simulink model "diagrama_completo"  (R2020b)
settings: Solver=VariableStepAuto  StartTime=0.0  StopTime=25  MaxStep=1e-4  RelTol=1e-4
model workspace (MAT data in the model file):
  Cts = 0.818
  Jeq = 5.65099476805e-06
  Ld = 0.0066
  Lls = 0.0008
  Lq = 0.0058
  Pp = 3
  Rs = 1.02
  Rts_amb = 146.7
  beq = 1.5e-05
  lambda_m = 0.01546
  r = 314.3008
  ws = 15000
  wsv = 30000
values from neighbouring files (symbols this model uses):
  ba = Jeq*n*wpos    (= 0.0113019895361)    [valores.m]
  kotheta = 3*pobs    (= 9600)    [valores.m]
  koTl = (pobs^3)    (= 32768000000)    [valores.m]
  kow = 3*(pobs^2)    (= 30720000)    [valores.m]
  ksa = ba*wpos    (= 9.04159162887)    [valores.m]
  ksia = ksa*wint    (= 2893.30932124)    [valores.m]
  R0 = Lls*pi    (= 4)    [valores.m]
  Rd = Ld*pi    (= 33)    [valores.m]
  Rq = Lq*pi    (= 29)    [valores.m]
undefined symbols (not defined in the file or in its folder): sigbuilder_block
(part 1 of 2)
settings Model: Creator=Matias  LastModifiedBy=Matias

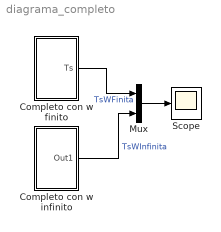
== system diagrama_completo ==
  Completo con w finito : Subsystem
  Completo con w infinito : Subsystem
  Mux : Mux  Inputs=2
  Scope : Scope
  wires:
  Completo con w finito/1(Ts) -> Mux/1  "TsWFinita"
  Completo con w infinito/1(Out1) -> Mux/2  "TsWInfinita"
  Mux/1 -> Scope/1

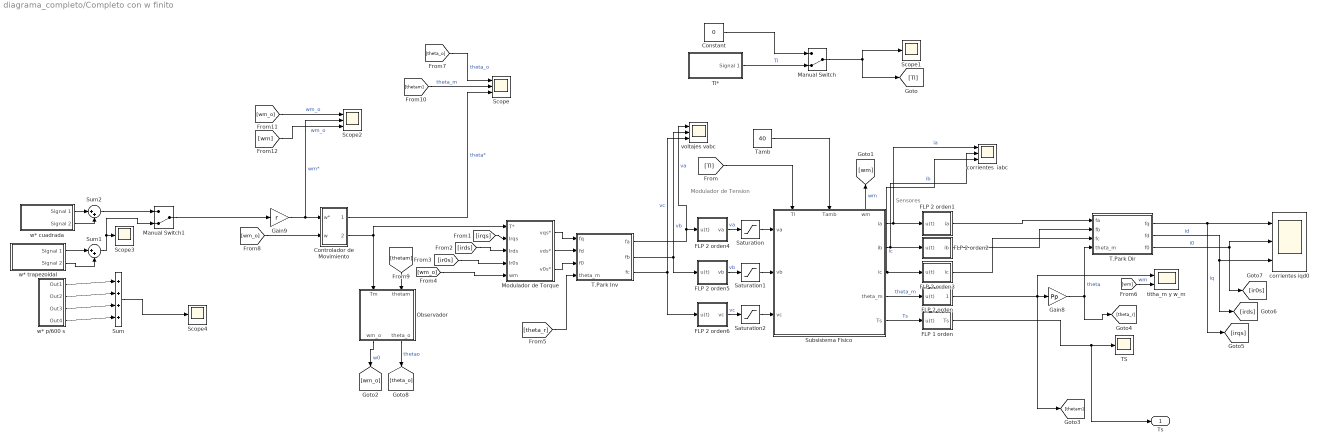
== system diagrama_completo/Completo con w finito ==
  note: Sensores
  note: Modulador de Tension
  Constant : Constant  Value=0
  Controlador de Movimiento : Subsystem
  FLP 1 orden : Subsystem
  FLP 2 orden : Subsystem
  FLP 2 orden1 : Subsystem
  FLP 2 orden2 : Subsystem
  FLP 2 orden3 : Subsystem
  FLP 2 orden4 : Subsystem
  FLP 2 orden5 : Subsystem
  FLP 2 orden6 : Subsystem
  Gain8 : Gain  Gain=Pp
  Gain9 : Gain  Gain=r
  Manual Switch : ManualSwitch  CurrentSetting=0
  Manual Switch1 : ManualSwitch  CurrentSetting=0
  Modulador de Torque : Subsystem
  Observador : Subsystem
  Saturation : Saturate  UpperLimit=19.59  LowerLimit=-19.59
  Saturation1 : Saturate  UpperLimit=19.59  LowerLimit=-19.59
  Saturation2 : Saturate  UpperLimit=19.59  LowerLimit=-19.59
  Scope : Scope  NumInputPorts=3
  Scope1 : Scope
  Scope2 : Scope  NumInputPorts=3
  Scope3 : Scope
  Scope4 : Scope
  Subsistema Fisico : Subsystem
      settings: PortSchema="{\"entries\":[{\"content\":{\"sides\":[{\"content\":{\"connectorIds\":[\"In1\",\"In2\",\"In3\"]},\"type\":\"ConnectorPlacement.EquallySpacedRectSide\",\"uuid\":\"428e53fe-c6d6-4999-95eb-db171c1d7752\"},{\"content\":{\"connectorIds\":[\"Out1\",\"Out2\",\"Out3\",\"Out4\",\"Out5\"],\"side\":\"RIGHT\"},\"type\":\"ConnectorPlacement.EquallySpacedRectSide\",\"uuid\":\"d3984cce-d898-4b9d-ab92-7967eebad5db\"},{\"content\":{\"connectorIds\":[\"In4\",\"In5\",\"Out6\"],\"side\":\"TOP\"},\"type\":\"ConnectorPlacement.EquallySpacedRectSide\",\"uuid\":\"4e08f4f3-ce82-4568-8c70-e26e1ed2ccd9\"},{\"content\":{\"connectorIds\":[],\"side\":\"BOTTOM\"},\"type\":\"ConnectorPlacement.EquallySpacedRectSide\",\"uuid\":\"f5359b7b-31c8-439d-9b4b-495d60398ac6\"},{\"content\":{\"connectorIds\":[],\"side\":\"HIDDEN\"},\"type\":\"ConnectorPlacement.EquallySpacedRectSide\",\"uuid\":\"fe5ef39c-0012-48bd-8627-0cf1abf153f6\"}]},\"type\":\"ConnectorPlacement.EquallySpacedConnector\",\"uuid\":\"3b2746a1-6d8c-49ea-8ba7-7e2e359e7a22\"}],\"packageUris\":[\"http://schema.mathworks.com/mf0/Connector/R2020b\"],\"version\":\"1.0\"}"
  Sum : Sum  Inputs=|+|+|+|+
  Sum1 : Sum  Inputs=|++
  Sum2 : Sum  Inputs=|++
  T.Park Dir : MATLAB Function  TreatAsAtomicUnit=on
  T.Park Inv : MATLAB Function  TreatAsAtomicUnit=on
  TS : Scope
  Tamb : Constant  Value=40
  Tl* : Subsystem  Tag=STV Subsys  LoadFcn=sigbuilder_block('load');  StartFcn=sigbuilder_block('start');  StopFcn=sigbuilder_block('stop');  ClipboardFcn=sigbuilder_block('clipboard');  mask(Sigbuilder block){tuvar=[0:10]}
      mask help: Simulink:masks:SigbuilderBlock_MD
      mask init:
      | if ~strcmp(get_param(bdroot(gcbh),'SimulationStatus'),'stopped') tuvar = sigbuilder_block('maskInit'); end
      settings: CopyFcn=sigbuilder_block('copy');  DeleteFcn=sigbuilder_block('delete');  ModelCloseFcn=sigbuilder_block('modelClose');  PreSaveFcn=sigbuilder_block('preSave');  PauseFcn=sigbuilder_block('pause');  ContinueFcn=sigbuilder_block('continue');  NameChangeFcn=sigbuilder_block('namechange');  OpenFcn=sigbuilder_block('open',[388.2 64.2 550.8 400.2 ]);  CloseFcn=sigbuilder_block('close');
      mask Display: plot(0, 0, 100, 100,[2, 2, 32, 32, 2], [68, 8, 8, 68, 68],[32, 2], [38, 38], [32, 19, 2],[53, 60, 44], [32, 17, 17, 2],[16, 16, 31, 31]);txt = getActiveGroup(gcbh);text(2, 100, txt,'verticalAlignment', 'top');
  corrientes  iabc : Scope  NumInputPorts=3
  corrientes iqd0 : Scope  NumInputPorts=3
  titha_m y w_m : Scope  NumInputPorts=2
  voltajes vabc : Scope  NumInputPorts=3
  w* cuadrada : Subsystem  Tag=STV Subsys  LoadFcn=sigbuilder_block('load');  StartFcn=sigbuilder_block('start');  StopFcn=sigbuilder_block('stop');  ClipboardFcn=sigbuilder_block('clipboard');  mask(Sigbuilder block){tuvar=[0:10]}
      mask help: Simulink:masks:SigbuilderBlock_MD
      mask init:
      | if ~strcmp(get_param(bdroot(gcbh),'SimulationStatus'),'stopped') tuvar = sigbuilder_block('maskInit'); end
      settings: CopyFcn=sigbuilder_block('copy');  DeleteFcn=sigbuilder_block('delete');  ModelCloseFcn=sigbuilder_block('modelClose');  PreSaveFcn=sigbuilder_block('preSave');  PauseFcn=sigbuilder_block('pause');  ContinueFcn=sigbuilder_block('continue');  NameChangeFcn=sigbuilder_block('namechange');  OpenFcn=sigbuilder_block('open',[5.4 36 1141.2 516.6 ]);  CloseFcn=sigbuilder_block('close');
      mask Display: plot(0, 0, 100, 100,[2, 2, 32, 32, 2], [68, 8, 8, 68, 68],[32, 2], [38, 38], [32, 19, 2],[53, 60, 44], [32, 17, 17, 2],[16, 16, 31, 31]);txt = getActiveGroup(gcbh);text(2, 100, txt,'verticalAlignment', 'top');
  w* p/600 s : Subsystem
  w* trapezoidal : Subsystem  Tag=STV Subsys  LoadFcn=sigbuilder_block('load');  StartFcn=sigbuilder_block('start');  StopFcn=sigbuilder_block('stop');  ClipboardFcn=sigbuilder_block('clipboard');  mask(Sigbuilder block){tuvar=[0:10]}
      mask help: Simulink:masks:SigbuilderBlock_MD
      mask init:
      | if ~strcmp(get_param(bdroot(gcbh),'SimulationStatus'),'stopped') tuvar = sigbuilder_block('maskInit'); end
      settings: CopyFcn=sigbuilder_block('copy');  DeleteFcn=sigbuilder_block('delete');  ModelCloseFcn=sigbuilder_block('modelClose');  PreSaveFcn=sigbuilder_block('preSave');  PauseFcn=sigbuilder_block('pause');  ContinueFcn=sigbuilder_block('continue');  NameChangeFcn=sigbuilder_block('namechange');  OpenFcn=sigbuilder_block('open',[5.4 36 1141.2 516.6 ]);  CloseFcn=sigbuilder_block('close');
      mask Display: plot(0, 0, 100, 100,[2, 2, 32, 32, 2], [68, 8, 8, 68, 68],[32, 2], [38, 38], [32, 19, 2],[53, 60, 44], [32, 17, 17, 2],[16, 16, 31, 31]);txt = getActiveGroup(gcbh);text(2, 100, txt,'verticalAlignment', 'top');
  Ts : Outport
  wires:
  T.Park Dir/2(fd) -> [irds], corrientes iqd0/3  "id"
  Modulador de Torque/2(vds*) -> T.Park Inv/2(fd)
  Subsistema Fisico/2(ib) -> FLP 2 orden2/1(u(t)), corrientes  iabc/2  "ib"
  FLP 2 orden6/1(vc) -> Saturation2/1  "vc"
  Gain8/1 -> T.Park Dir/4(theta_m), [theta_r]  "theta"
  Saturation1/1 -> Subsistema Fisico/2(vb)
  [thetam] -> Observador/2(thetam)
  [wm_o] -> Modulador de Torque/5(wm)
  Saturation/1 -> Subsistema Fisico/1(va)
  Sum/1 -> Scope4/1
  w* cuadrada/1(Signal 1) -> Sum2/1
  Subsistema Fisico/3(ic) -> FLP 2 orden3/1(u(t)), corrientes  iabc/3  "ic"
  FLP 2 orden4/1(va) -> Saturation/1  "va"
  w* p/600 s/2(Out2) -> Sum/2
  Subsistema Fisico/5(Ts) -> FLP 1 orden/1(u(t))  "Ts"
  T.Park Inv/1(fa) -> FLP 2 orden4/1(u(t)), voltajes vabc/1  "va"
  Manual Switch1/1 -> Gain9/1
  FLP 2 orden/1(theta) -> [thetam], titha_m y w_m/1, Gain8/1
  Tl*/1(Signal 1) -> Manual Switch/2  "Tl"
  Modulador de Torque/1(vqs*) -> T.Park Inv/1(fq)
  Saturation2/1 -> Subsistema Fisico/3(vc)
  w* trapezoidal/1(Signal 1) -> Sum1/1
  [irqs] -> Modulador de Torque/2(Irqs)
  Subsistema Fisico/1(ia) -> corrientes  iabc/1, FLP 2 orden1/1(u(t))  "ia"
  Sum1/1 -> Manual Switch1/2, Scope3/1
  FLP 2 orden2/1(ib) -> T.Park Dir/2(fb)
  [irds] -> Modulador de Torque/3(Irds)
  Tamb/1 -> Subsistema Fisico/5(Tamb)
  Constant/1 -> Manual Switch/1
  [theta_r] -> T.Park Inv/4(theta_m)
  T.Park Dir/1(fq) -> [irqs], corrientes iqd0/1  "iq"
  [ir0s] -> Modulador de Torque/4(Ir0s)
  [wm_o] -> Scope2/1  "wm_o"
  Subsistema Fisico/4(theta_m) -> FLP 2 orden/1(u(t))  "theta_m"
  [wm_o] -> Controlador de Movimiento/2(w)
  [Tl] -> Subsistema Fisico/4(Tl)
  T.Park Dir/3(f0) -> [ir0s], corrientes iqd0/2  "i0"
  Sum2/1 -> Manual Switch1/1
  Observador/1(wm_o) -> [wm_o]  "w0"
  w* p/600 s/1(Out1) -> Sum/1
  [wm] -> titha_m y w_m/2  "wm"
  Gain9/1 -> Scope2/2, Controlador de Movimiento/1(w*)  "wm*"
  Observador/2(theta_o) -> [theta_o]  "thetao"
  Controlador de Movimiento/1(Theta*) -> Scope/3  "theta*"
  w* trapezoidal/2(Signal 2) -> Sum1/2
  [theta_o] -> Scope/1  "theta_o"
  Manual Switch/1 -> [Tl], Scope1/1
  [thetam] -> Scope/2  "theta_m"
  Subsistema Fisico/6(wm) -> [wm]  "wm"
  Modulador de Torque/3(v0s*) -> T.Park Inv/3(f0)
  FLP 2 orden3/1(ic) -> T.Park Dir/3(fc)
  w* p/600 s/3(Out3) -> Sum/3
  FLP 1 orden/1(Ts) -> Ts/1, TS/1
  Controlador de Movimiento/2(Tm*') -> Modulador de Torque/1(T*), Observador/1(Tm)
  w* cuadrada/2(Signal 2) -> Sum2/2
  T.Park Inv/3(fc) -> voltajes vabc/3, FLP 2 orden6/1(u(t))  "vc"
  T.Park Inv/2(fb) -> FLP 2 orden5/1(u(t)), voltajes vabc/2  "vb"
  FLP 2 orden1/1(ia) -> T.Park Dir/1(fa)
  w* p/600 s/4(Out4) -> Sum/4
  [wm] -> Scope2/3  "wm_o"
  FLP 2 orden5/1(vb) -> Saturation1/1  "vb"

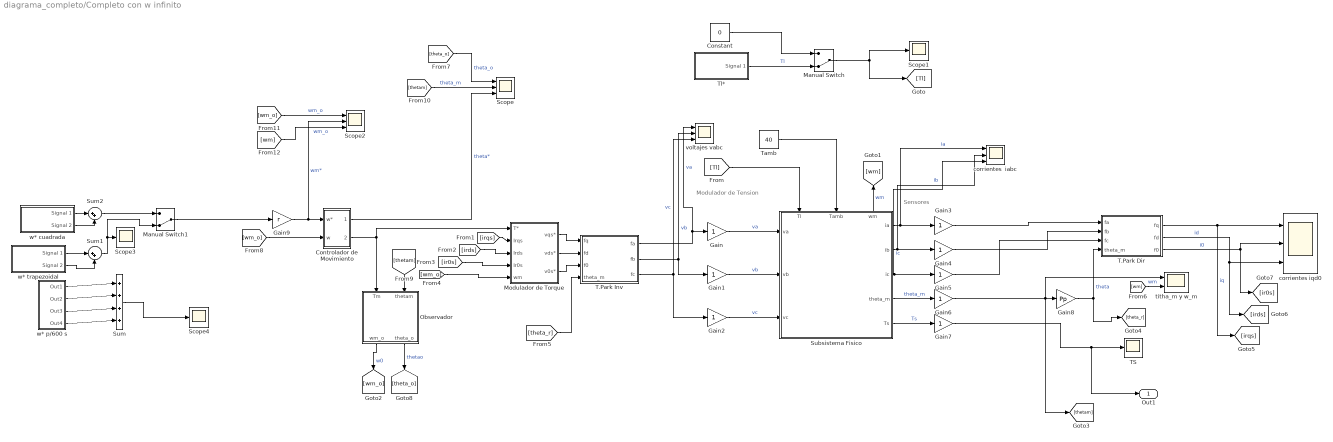
== system diagrama_completo/Completo con w infinito ==
  note: Sensores
  note: Modulador de Tension
  Constant : Constant  Value=0
  Controlador de Movimiento : Subsystem
  Gain{,1..7} (8 alike) : Gain
  Gain8 : Gain  Gain=Pp
  Gain9 : Gain  Gain=r
  Manual Switch : ManualSwitch  CurrentSetting=0
  Manual Switch1 : ManualSwitch  CurrentSetting=0
  Modulador de Torque : Subsystem
  Observador : Subsystem
  Scope : Scope  NumInputPorts=3
  Scope1 : Scope
  Scope2 : Scope  NumInputPorts=3
  Scope3 : Scope
  Scope4 : Scope
  Subsistema Fisico : Subsystem
      settings: PortSchema="{\"entries\":[{\"content\":{\"sides\":[{\"content\":{\"connectorIds\":[\"In1\",\"In2\",\"In3\"]},\"type\":\"ConnectorPlacement.EquallySpacedRectSide\",\"uuid\":\"428e53fe-c6d6-4999-95eb-db171c1d7752\"},{\"content\":{\"connectorIds\":[\"Out1\",\"Out2\",\"Out3\",\"Out4\",\"Out5\"],\"side\":\"RIGHT\"},\"type\":\"ConnectorPlacement.EquallySpacedRectSide\",\"uuid\":\"d3984cce-d898-4b9d-ab92-7967eebad5db\"},{\"content\":{\"connectorIds\":[\"In4\",\"In5\",\"Out6\"],\"side\":\"TOP\"},\"type\":\"ConnectorPlacement.EquallySpacedRectSide\",\"uuid\":\"4e08f4f3-ce82-4568-8c70-e26e1ed2ccd9\"},{\"content\":{\"connectorIds\":[],\"side\":\"BOTTOM\"},\"type\":\"ConnectorPlacement.EquallySpacedRectSide\",\"uuid\":\"f5359b7b-31c8-439d-9b4b-495d60398ac6\"},{\"content\":{\"connectorIds\":[],\"side\":\"HIDDEN\"},\"type\":\"ConnectorPlacement.EquallySpacedRectSide\",\"uuid\":\"fe5ef39c-0012-48bd-8627-0cf1abf153f6\"}]},\"type\":\"ConnectorPlacement.EquallySpacedConnector\",\"uuid\":\"3b2746a1-6d8c-49ea-8ba7-7e2e359e7a22\"}],\"packageUris\":[\"http://schema.mathworks.com/mf0/Connector/R2020b\"],\"version\":\"1.0\"}"
  Sum : Sum  Inputs=|+|+|+|+
  Sum1 : Sum  Inputs=|++
  Sum2 : Sum  Inputs=|++
  T.Park Dir : MATLAB Function  TreatAsAtomicUnit=on
  T.Park Inv : MATLAB Function  TreatAsAtomicUnit=on
  TS : Scope
  Tamb : Constant  Value=40
  Tl* : Subsystem  Tag=STV Subsys  LoadFcn=sigbuilder_block('load');  StartFcn=sigbuilder_block('start');  StopFcn=sigbuilder_block('stop');  ClipboardFcn=sigbuilder_block('clipboard');  mask(Sigbuilder block){tuvar=[0:10]}
      mask help: Simulink:masks:SigbuilderBlock_MD
      mask init:
      | if ~strcmp(get_param(bdroot(gcbh),'SimulationStatus'),'stopped') tuvar = sigbuilder_block('maskInit'); end
      settings: CopyFcn=sigbuilder_block('copy');  DeleteFcn=sigbuilder_block('delete');  ModelCloseFcn=sigbuilder_block('modelClose');  PreSaveFcn=sigbuilder_block('preSave');  PauseFcn=sigbuilder_block('pause');  ContinueFcn=sigbuilder_block('continue');  NameChangeFcn=sigbuilder_block('namechange');  OpenFcn=sigbuilder_block('open',[388.2 64.2 550.8 400.2 ]);  CloseFcn=sigbuilder_block('close');
      mask Display: plot(0, 0, 100, 100,[2, 2, 32, 32, 2], [68, 8, 8, 68, 68],[32, 2], [38, 38], [32, 19, 2],[53, 60, 44], [32, 17, 17, 2],[16, 16, 31, 31]);txt = getActiveGroup(gcbh);text(2, 100, txt,'verticalAlignment', 'top');
  corrientes  iabc : Scope  NumInputPorts=3
  corrientes iqd0 : Scope  NumInputPorts=3
  titha_m y w_m : Scope  NumInputPorts=2
  voltajes vabc : Scope  NumInputPorts=3
  w* cuadrada : Subsystem  Tag=STV Subsys  LoadFcn=sigbuilder_block('load');  StartFcn=sigbuilder_block('start');  StopFcn=sigbuilder_block('stop');  ClipboardFcn=sigbuilder_block('clipboard');  mask(Sigbuilder block){tuvar=[0:10]}
      mask help: Simulink:masks:SigbuilderBlock_MD
      mask init:
      | if ~strcmp(get_param(bdroot(gcbh),'SimulationStatus'),'stopped') tuvar = sigbuilder_block('maskInit'); end
      settings: CopyFcn=sigbuilder_block('copy');  DeleteFcn=sigbuilder_block('delete');  ModelCloseFcn=sigbuilder_block('modelClose');  PreSaveFcn=sigbuilder_block('preSave');  PauseFcn=sigbuilder_block('pause');  ContinueFcn=sigbuilder_block('continue');  NameChangeFcn=sigbuilder_block('namechange');  OpenFcn=sigbuilder_block('open',[5.4 36 1141.2 516.6 ]);  CloseFcn=sigbuilder_block('close');
      mask Display: plot(0, 0, 100, 100,[2, 2, 32, 32, 2], [68, 8, 8, 68, 68],[32, 2], [38, 38], [32, 19, 2],[53, 60, 44], [32, 17, 17, 2],[16, 16, 31, 31]);txt = getActiveGroup(gcbh);text(2, 100, txt,'verticalAlignment', 'top');
  w* p/600 s : Subsystem
  w* trapezoidal : Subsystem  Tag=STV Subsys  LoadFcn=sigbuilder_block('load');  StartFcn=sigbuilder_block('start');  StopFcn=sigbuilder_block('stop');  ClipboardFcn=sigbuilder_block('clipboard');  mask(Sigbuilder block){tuvar=[0:10]}
      mask help: Simulink:masks:SigbuilderBlock_MD
      mask init:
      | if ~strcmp(get_param(bdroot(gcbh),'SimulationStatus'),'stopped') tuvar = sigbuilder_block('maskInit'); end
      settings: CopyFcn=sigbuilder_block('copy');  DeleteFcn=sigbuilder_block('delete');  ModelCloseFcn=sigbuilder_block('modelClose');  PreSaveFcn=sigbuilder_block('preSave');  PauseFcn=sigbuilder_block('pause');  ContinueFcn=sigbuilder_block('continue');  NameChangeFcn=sigbuilder_block('namechange');  OpenFcn=sigbuilder_block('open',[5.4 36 1141.2 516.6 ]);  CloseFcn=sigbuilder_block('close');
      mask Display: plot(0, 0, 100, 100,[2, 2, 32, 32, 2], [68, 8, 8, 68, 68],[32, 2], [38, 38], [32, 19, 2],[53, 60, 44], [32, 17, 17, 2],[16, 16, 31, 31]);txt = getActiveGroup(gcbh);text(2, 100, txt,'verticalAlignment', 'top');
  Out1 : Outport
  wires:
  [theta_r] -> T.Park Inv/4(theta_m)
  w* p/600 s/4(Out4) -> Sum/4
  [wm_o] -> Controlador de Movimiento/2(w)
  Gain8/1 -> T.Park Dir/4(theta_m), [theta_r]  "theta"
  Manual Switch1/1 -> Gain9/1
  Controlador de Movimiento/1(Theta*) -> Scope/3  "theta*"
  Subsistema Fisico/3(ic) -> Gain5/1, corrientes  iabc/3  "ic"
  T.Park Dir/1(fq) -> [irqs], corrientes iqd0/1  "iq"
  Gain/1 -> Subsistema Fisico/1(va)  "va"
  T.Park Inv/2(fb) -> Gain1/1, voltajes vabc/2  "vb"
  Subsistema Fisico/2(ib) -> Gain4/1, corrientes  iabc/2  "ib"
  Gain6/1 -> [thetam], titha_m y w_m/1, Gain8/1
  w* cuadrada/2(Signal 2) -> Sum2/2
  T.Park Inv/1(fa) -> Gain/1, voltajes vabc/1  "va"
  T.Park Dir/2(fd) -> [irds], corrientes iqd0/3  "id"
  Modulador de Torque/1(vqs*) -> T.Park Inv/1(fq)
  Modulador de Torque/3(v0s*) -> T.Park Inv/3(f0)
  Gain3/1 -> T.Park Dir/1(fa)
  Observador/2(theta_o) -> [theta_o]  "thetao"
  Gain7/1 -> Out1/1, TS/1
  Subsistema Fisico/4(theta_m) -> Gain6/1  "theta_m"
  Controlador de Movimiento/2(Tm*') -> Modulador de Torque/1(T*), Observador/1(Tm)
  w* p/600 s/2(Out2) -> Sum/2
  Gain9/1 -> Scope2/2, Controlador de Movimiento/1(w*)  "wm*"
  Sum1/1 -> Manual Switch1/2, Scope3/1
  [theta_o] -> Scope/1  "theta_o"
  [Tl] -> Subsistema Fisico/4(Tl)
  [thetam] -> Scope/2  "theta_m"
  w* p/600 s/1(Out1) -> Sum/1
  w* trapezoidal/1(Signal 1) -> Sum1/1
  w* cuadrada/1(Signal 1) -> Sum2/1
  Tl*/1(Signal 1) -> Manual Switch/2  "Tl"
  T.Park Dir/3(f0) -> [ir0s], corrientes iqd0/2  "i0"
  w* p/600 s/3(Out3) -> Sum/3
  Gain5/1 -> T.Park Dir/3(fc)
  Gain2/1 -> Subsistema Fisico/3(vc)  "vc"
  [irqs] -> Modulador de Torque/2(Irqs)
  T.Park Inv/3(fc) -> Gain2/1, voltajes vabc/3  "vc"
  [wm_o] -> Modulador de Torque/5(wm)
  [irds] -> Modulador de Torque/3(Irds)
  [thetam] -> Observador/2(thetam)
  [wm] -> Scope2/3  "wm_o"
  Subsistema Fisico/6(wm) -> [wm]  "wm"
  Sum2/1 -> Manual Switch1/1
  [wm] -> titha_m y w_m/2  "wm"
  w* trapezoidal/2(Signal 2) -> Sum1/2
  Manual Switch/1 -> [Tl], Scope1/1
  Constant/1 -> Manual Switch/1
  Sum/1 -> Scope4/1
  Subsistema Fisico/5(Ts) -> Gain7/1  "Ts"
  Subsistema Fisico/1(ia) -> Gain3/1, corrientes  iabc/1  "ia"
  Tamb/1 -> Subsistema Fisico/5(Tamb)
  [ir0s] -> Modulador de Torque/4(Ir0s)
  Modulador de Torque/2(vds*) -> T.Park Inv/2(fd)
  Gain4/1 -> T.Park Dir/2(fb)
  Gain1/1 -> Subsistema Fisico/2(vb)  "vb"
  Observador/1(wm_o) -> [wm_o]  "w0"
  [wm_o] -> Scope2/1  "wm_o"

== system diagrama_completo/Completo con w finito/Controlador de Movimiento ==
  w* : Inport
  w : Inport  Port=2
  Gain : Gain  Gain=ba
  Gain1 : Gain  Gain=ksa
  Gain2 : Gain  Gain=ksia
  Integrator : Integrator
  Integrator1 : Integrator
  Integrator2 : Integrator
  Sum : Sum  Inputs=|+++
  Sum1 : Sum  Inputs=|+-
  Theta* : Outport
  Tm*' : Outport  Port=2
  wires:
  w*/1 -> Integrator2/1, Sum1/1
  w/1 -> Sum1/2
  Sum1/1 -> Integrator/1, Gain/1  "ew"
  Sum/1 -> Tm*'/1
  Gain/1 -> Sum/3
  Gain1/1 -> Sum/2
  Integrator1/1 -> Gain2/1  "etheta/s"
  Integrator/1 -> Integrator1/1, Gain1/1  "etheta"
  Gain2/1 -> Sum/1
  Integrator2/1 -> Theta*/1  "etheta"

== system diagrama_completo/Completo con w finito/FLP 1 orden ==
  u(t) : Inport
  Gain : Gain
  Gain1 : Gain
  Gain2 : Gain  Gain=1/2
  Integrator1 : Integrator  InitialCondition=40
  Sum : Sum  Inputs=|+|-
  Ts : Outport
  wires:
  u(t)/1 -> Gain/1
  Integrator1/1 -> Ts/1, Gain1/1  "x1"
  Gain/1 -> Sum/1
  Gain1/1 -> Sum/2
  Sum/1 -> Gain2/1  "d(x1)"
  Gain2/1 -> Integrator1/1

== system diagrama_completo/Completo con w finito/FLP 2 orden ==
  u(t) : Inport
  Gain : Gain  Gain=ws^2
  Gain1 : Gain  Gain=2*ws*1
  Gain2 : Gain  Gain=(ws^2)
  Integrator : Integrator
  Integrator1 : Integrator
  Sum : Sum  Inputs=|+|-|-
  theta : Outport
  wires:
  u(t)/1 -> Gain/1
  Integrator1/1 -> Gain1/1, Integrator/1  "x2"
  Integrator/1 -> Gain2/1, theta/1  "x1"
  Gain/1 -> Sum/1
  Sum/1 -> Integrator1/1  "d(x2)"
  Gain1/1 -> Sum/3
  Gain2/1 -> Sum/2

== system diagrama_completo/Completo con w finito/FLP 2 orden1 ==
  u(t) : Inport
  Gain : Gain  Gain=ws^2
  Gain1 : Gain  Gain=2*ws*1
  Gain2 : Gain  Gain=(ws^2)
  Integrator : Integrator
  Integrator1 : Integrator
  Sum : Sum  Inputs=|+|-|-
  ia : Outport
  wires:
  u(t)/1 -> Gain/1
  Integrator1/1 -> Gain1/1, Integrator/1  "x2"
  Integrator/1 -> Gain2/1, ia/1  "x1"
  Gain/1 -> Sum/1
  Sum/1 -> Integrator1/1  "d(x2)"
  Gain1/1 -> Sum/3
  Gain2/1 -> Sum/2

== system diagrama_completo/Completo con w finito/FLP 2 orden2 ==
  u(t) : Inport
  Gain : Gain  Gain=ws^2
  Gain1 : Gain  Gain=2*ws*1
  Gain2 : Gain  Gain=(ws^2)
  Integrator : Integrator
  Integrator1 : Integrator
  Sum : Sum  Inputs=|+|-|-
  ib : Outport
  wires:
  u(t)/1 -> Gain/1
  Integrator1/1 -> Gain1/1, Integrator/1  "x2"
  Integrator/1 -> Gain2/1, ib/1  "x1"
  Gain/1 -> Sum/1
  Sum/1 -> Integrator1/1  "d(x2)"
  Gain1/1 -> Sum/3
  Gain2/1 -> Sum/2

== system diagrama_completo/Completo con w finito/FLP 2 orden3 ==
  u(t) : Inport
  Gain : Gain  Gain=ws^2
  Gain1 : Gain  Gain=2*ws*1
  Gain2 : Gain  Gain=(ws^2)
  Integrator : Integrator
  Integrator1 : Integrator
  Sum : Sum  Inputs=|+|-|-
  ic : Outport
  wires:
  u(t)/1 -> Gain/1
  Integrator1/1 -> Gain1/1, Integrator/1  "x2"
  Integrator/1 -> Gain2/1, ic/1  "x1"
  Gain/1 -> Sum/1
  Sum/1 -> Integrator1/1  "d(x2)"
  Gain1/1 -> Sum/3
  Gain2/1 -> Sum/2

== system diagrama_completo/Completo con w finito/FLP 2 orden4 ==
  u(t) : Inport
  Gain : Gain  Gain=wsv^2
  Gain1 : Gain  Gain=2*wsv*1
  Gain2 : Gain  Gain=(wsv^2)
  Integrator : Integrator
  Integrator1 : Integrator
  Sum : Sum  Inputs=|+|-|-
  va : Outport
  wires:
  u(t)/1 -> Gain/1
  Integrator1/1 -> Gain1/1, Integrator/1  "x2"
  Integrator/1 -> Gain2/1, va/1  "x1"
  Gain/1 -> Sum/1
  Sum/1 -> Integrator1/1  "d(x2)"
  Gain1/1 -> Sum/3
  Gain2/1 -> Sum/2

== system diagrama_completo/Completo con w finito/FLP 2 orden5 ==
  u(t) : Inport
  Gain : Gain  Gain=wsv^2
  Gain1 : Gain  Gain=2*wsv*1
  Gain2 : Gain  Gain=(wsv^2)
  Integrator : Integrator
  Integrator1 : Integrator
  Sum : Sum  Inputs=|+|-|-
  vb : Outport
  wires:
  u(t)/1 -> Gain/1
  Integrator1/1 -> Gain1/1, Integrator/1  "x2"
  Integrator/1 -> Gain2/1, vb/1  "x1"
  Gain/1 -> Sum/1
  Sum/1 -> Integrator1/1  "d(x2)"
  Gain1/1 -> Sum/3
  Gain2/1 -> Sum/2

== system diagrama_completo/Completo con w finito/FLP 2 orden6 ==
  u(t) : Inport
  Gain : Gain  Gain=wsv^2
  Gain1 : Gain  Gain=2*wsv*1
  Gain2 : Gain  Gain=(wsv^2)
  Integrator : Integrator
  Integrator1 : Integrator
  Sum : Sum  Inputs=|+|-|-
  vc : Outport
  wires:
  u(t)/1 -> Gain/1
  Integrator1/1 -> Gain1/1, Integrator/1  "x2"
  Integrator/1 -> Gain2/1, vc/1  "x1"
  Gain/1 -> Sum/1
  Sum/1 -> Integrator1/1  "d(x2)"
  Gain1/1 -> Sum/3
  Gain2/1 -> Sum/2

== system diagrama_completo/Completo con w finito/Modulador de Torque ==
  T* : Inport
  Irqs : Inport  Port=2
  Irds : Inport  Port=3
  Ir0s : Inport  Port=4
  wm : Inport  Port=5
  Constant : Constant  Value=0
  Constant1 : Constant  Value=0
  Control de Corriente : Subsystem
  Gain3 : Gain  Gain=beq
  Gain9 : Gain  Gain=1/((3/2)*Pp*lambda_m)
  Sum : Sum  Inputs=|++
  vqs* : Outport
  vds* : Outport  Port=2
  v0s* : Outport  Port=3
  wires:
  Control de Corriente/2(vds*) -> vds*/1
  Irds/1 -> Control de Corriente/5(Irds)
  Gain9/1 -> Control de Corriente/1(Irqs*)
  Ir0s/1 -> Control de Corriente/6(Ir0s)
  Constant/1 -> Control de Corriente/3(Ir0s*)
  Control de Corriente/3(v0s*) -> v0s*/1
  Constant1/1 -> Control de Corriente/2(Irds*)
  Control de Corriente/1(vqs*) -> vqs*/1
  Irqs/1 -> Control de Corriente/4(Irqs)
  Sum/1 -> Gain9/1
  T*/1 -> Sum/1
  wm/1 -> Gain3/1, Control de Corriente/7(wm)
  Gain3/1 -> Sum/2

== system diagrama_completo/Completo con w finito/Observador ==
  Tm : Inport
  thetam : Inport  Port=2
  Gain : Gain  Gain=kow
  Gain1 : Gain  Gain=koTl
  Gain2 : Gain  Gain=kotheta
  Gain9 : Gain  Gain=1/Jeq
  Integrator : Integrator
  Integrator1 : Integrator
  Integrator2 : Integrator
  Sum1 : Sum  Inputs=+|+|+
  Sum2 : Sum  Inputs=+|+
  Sum3 : Sum  Inputs=|+-
  wm_o : Outport
  theta_o : Outport  Port=2
  wires:
  Tm/1 -> Gain9/1
  Integrator1/1 -> theta_o/1, Sum3/2  "theta_o"
  Sum1/1 -> Integrator/1
  Sum2/1 -> wm_o/1, Integrator1/1
  thetam/1 -> Sum3/1
  Sum3/1 -> Gain2/1, Integrator2/1, Gain/1  "eo"
  Gain/1 -> Sum1/1
  Integrator/1 -> Sum2/2
  Gain2/1 -> Sum2/1
  Integrator2/1 -> Gain1/1
  Gain9/1 -> Sum1/3
  Gain1/1 -> Sum1/2

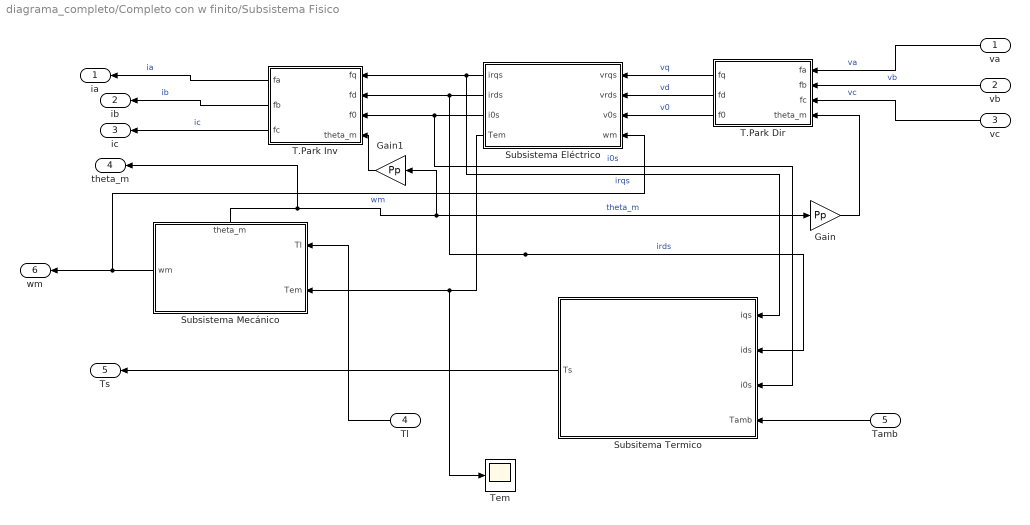
== system diagrama_completo/Completo con w finito/Subsistema Fisico ==
  va : Inport
  vb : Inport  Port=2
  vc : Inport  Port=3
  Tl : Inport  Port=4
  Tamb : Inport  Port=5
  Gain : Gain  Gain=Pp
  Gain1 : Gain  Gain=Pp
  Subsistema Eléctrico : Subsystem
  Subsistema Mecánico : Subsystem
      settings: PortSchema="{\"entries\":[{\"content\":{\"sides\":[{\"content\":{\"connectorIds\":[\"In1\",\"In2\"]},\"type\":\"ConnectorPlacement.EquallySpacedRectSide\",\"uuid\":\"ee0e19e9-1195-452b-ab3d-8be3dd040414\"},{\"content\":{\"connectorIds\":[\"Out1\"],\"side\":\"RIGHT\"},\"type\":\"ConnectorPlacement.EquallySpacedRectSide\",\"uuid\":\"524e54e6-4967-4b42-ae12-58774e9397a0\"},{\"content\":{\"connectorIds\":[\"Out2\"],\"side\":\"TOP\"},\"type\":\"ConnectorPlacement.EquallySpacedRectSide\",\"uuid\":\"fab71378-68cb-4446-b02c-df48705d1789\"},{\"content\":{\"connectorIds\":[],\"side\":\"HIDDEN\"},\"type\":\"ConnectorPlacement.EquallySpacedRectSide\",\"uuid\":\"eea92cb8-3517-43ef-96fe-10b46f054d59\"}]},\"type\":\"ConnectorPlacement.EquallySpacedConnector\",\"uuid\":\"156d3ac5-e5c7-4248-8590-4f82c7370a76\"}],\"packageUris\":[\"http://schema.mathworks.com/mf0/Connector/R2020b\"],\"version\":\"1.0\"}"
  Subsitema Termico : Subsystem
  T.Park Dir : MATLAB Function  TreatAsAtomicUnit=on
  T.Park Inv : MATLAB Function  TreatAsAtomicUnit=on
  Tem : Scope
  ia : Outport
  ib : Outport  Port=2
  ic : Outport  Port=3
  theta_m : Outport  Port=4
  Ts : Outport  Port=5
  wm : Outport  Port=6
  wires:
  Subsitema Termico/1(Ts) -> Ts/1
  Tl/1 -> Subsistema Mecánico/1(Tl)
  T.Park Inv/3(fc) -> ic/1  "ic"
  vb/1 -> T.Park Dir/2(fb)  "vb"
  Tamb/1 -> Subsitema Termico/4(Tamb)
  T.Park Inv/1(fa) -> ia/1  "ia"
  Subsistema Mecánico/1(wm) -> Subsistema Eléctrico/4(wm), wm/1  "wm"
  T.Park Dir/1(fq) -> Subsistema Eléctrico/1(vrqs)  "vq"
  Subsistema Eléctrico/3(i0s) -> Subsitema Termico/3(i0s), T.Park Inv/3(f0)  "i0s"
  Subsistema Eléctrico/1(irqs) -> Subsitema Termico/1(iqs), T.Park Inv/1(fq)  "irqs"
  Subsistema Eléctrico/2(irds) -> Subsitema Termico/2(ids), T.Park Inv/2(fd)  "irds"
  T.Park Dir/3(f0) -> Subsistema Eléctrico/3(v0s)  "v0"
  T.Park Dir/2(fd) -> Subsistema Eléctrico/2(vrds)  "vd"
  vc/1 -> T.Park Dir/3(fc)  "vc"
  T.Park Inv/2(fb) -> ib/1  "ib"
  Subsistema Mecánico/2(theta_m) -> theta_m/1, Gain1/1, Gain/1  "theta_m"
  va/1 -> T.Park Dir/1(fa)  "va"
  Subsistema Eléctrico/4(Tem) -> Tem/1, Subsistema Mecánico/2(Tem)
  Gain/1 -> T.Park Dir/4(theta_m)
  Gain1/1 -> T.Park Inv/4(theta_m)

== system diagrama_completo/Completo con w finito/Tl* ==
  Demux : Demux  Tag=STV Demux  Outputs=1
      settings: DisplayOption=none
  FromWs : FromWorkspace  Tag=STV FromWs  VariableName=tuvar
      SigBuilderData=|
      | common.afterFinalStr = 'Extrapolate'
      | common.sampleTime = 0
      | dataSet.timeRange = [0 25]
      | dataSet.name = 'Group 1'
      | sbobj.Groups.Name = 'Group 1'
      | sbobj.Groups.Signals.Name = 'Signal 1'
      | sbobj.Groups.Signals.XData = [0 1 1 25]
      | sbobj.Groups.Signals.YData = [0 0 6.28 6.28]
      | sbobj.Groups.TimeRange = [0 25]
  Signal 1 : Outport  Tag=STV Outport
  wires:
  Demux/1 -> Signal 1/1
  FromWs/1 -> Demux/1

== system diagrama_completo/Completo con w finito/w* cuadrada ==
  Demux : Demux  Tag=STV Demux  Outputs=2
      settings: DisplayOption=none
  FromWs : FromWorkspace  Tag=STV FromWs  VariableName=tuvar
      SigBuilderData=|
      | common.afterFinalStr = 'Extrapolate'
      | common.sampleTime = 0
      | dataSet.timeRange = [0 25]
      | dataSet.name = 'Group 1'
      | sbobj.Groups.Name = 'Group 1'
      | sbobj.Groups.Signals(1).Name = 'Signal 1'
      | sbobj.Groups.Signals(1).XData = [0 5 5 10 10 25]
      | sbobj.Groups.Signals(1).YData = [0 0 1.25663706144 1.25663706144 0 0]
      | sbobj.Groups.Signals(2).Name = 'Signal 2'
      | sbobj.Groups.Signals(2).XData = [0 15 15 20 20 25]
      | sbobj.Groups.Signals(2).YData = [0 0 -1.25663706144 -1.25663706144 0 0]
      | sbobj.Groups.TimeRange = [0 25]
  Signal 1 : Outport  Tag=STV Outport
  Signal 2 : Outport  Tag=STV Outport  Port=2
  wires:
  FromWs/1 -> Demux/1
  Demux/1 -> Signal 1/1
  Demux/2 -> Signal 2/1

== system diagrama_completo/Completo con w finito/w* p//600 s ==
  Sum{3..6} (4 alike) : Sum  Inputs=|+++++++++++++++
  w* trapezoidal1 : Subsystem  Tag=STV Subsys  LoadFcn=sigbuilder_block('load');  StartFcn=sigbuilder_block('start');  StopFcn=sigbuilder_block('stop');  ClipboardFcn=sigbuilder_block('clipboard');  mask(Sigbuilder block){tuvar=[0:10]}
      mask help: Simulink:masks:SigbuilderBlock_MD
      mask init:
      | if ~strcmp(get_param(bdroot(gcbh),'SimulationStatus'),'stopped') tuvar = sigbuilder_block('maskInit'); end
      settings: CopyFcn=sigbuilder_block('copy');  DeleteFcn=sigbuilder_block('delete');  ModelCloseFcn=sigbuilder_block('modelClose');  PreSaveFcn=sigbuilder_block('preSave');  PauseFcn=sigbuilder_block('pause');  ContinueFcn=sigbuilder_block('continue');  NameChangeFcn=sigbuilder_block('namechange');  OpenFcn=sigbuilder_block('open',[5.4 36 1141.2 516.6 ]);  CloseFcn=sigbuilder_block('close');
      mask Display: plot(0, 0, 100, 100,[2, 2, 32, 32, 2], [68, 8, 8, 68, 68],[32, 2], [38, 38], [32, 19, 2],[53, 60, 44], [32, 17, 17, 2],[16, 16, 31, 31]);txt = getActiveGroup(gcbh);text(2, 100, txt,'verticalAlignment', 'top');
  w* trapezoidal2 : Subsystem  Tag=STV Subsys  LoadFcn=sigbuilder_block('load');  StartFcn=sigbuilder_block('start');  StopFcn=sigbuilder_block('stop');  ClipboardFcn=sigbuilder_block('clipboard');  mask(Sigbuilder block){tuvar=[0:10]}
      mask help: Simulink:masks:SigbuilderBlock_MD
      mask init:
      | if ~strcmp(get_param(bdroot(gcbh),'SimulationStatus'),'stopped') tuvar = sigbuilder_block('maskInit'); end
      settings: CopyFcn=sigbuilder_block('copy');  DeleteFcn=sigbuilder_block('delete');  ModelCloseFcn=sigbuilder_block('modelClose');  PreSaveFcn=sigbuilder_block('preSave');  PauseFcn=sigbuilder_block('pause');  ContinueFcn=sigbuilder_block('continue');  NameChangeFcn=sigbuilder_block('namechange');  OpenFcn=sigbuilder_block('open',[5.4 36 1141.2 516.6 ]);  CloseFcn=sigbuilder_block('close');
      mask Display: plot(0, 0, 100, 100,[2, 2, 32, 32, 2], [68, 8, 8, 68, 68],[32, 2], [38, 38], [32, 19, 2],[53, 60, 44], [32, 17, 17, 2],[16, 16, 31, 31]);txt = getActiveGroup(gcbh);text(2, 100, txt,'verticalAlignment', 'top');
  w* trapezoidal3 : Subsystem  Tag=STV Subsys  LoadFcn=sigbuilder_block('load');  StartFcn=sigbuilder_block('start');  StopFcn=sigbuilder_block('stop');  ClipboardFcn=sigbuilder_block('clipboard');  mask(Sigbuilder block){tuvar=[0:10]}
      mask help: Simulink:masks:SigbuilderBlock_MD
      mask init:
      | if ~strcmp(get_param(bdroot(gcbh),'SimulationStatus'),'stopped') tuvar = sigbuilder_block('maskInit'); end
      settings: CopyFcn=sigbuilder_block('copy');  DeleteFcn=sigbuilder_block('delete');  ModelCloseFcn=sigbuilder_block('modelClose');  PreSaveFcn=sigbuilder_block('preSave');  PauseFcn=sigbuilder_block('pause');  ContinueFcn=sigbuilder_block('continue');  NameChangeFcn=sigbuilder_block('namechange');  OpenFcn=sigbuilder_block('open',[5.4 36 1141.2 516.6 ]);  CloseFcn=sigbuilder_block('close');
      mask Display: plot(0, 0, 100, 100,[2, 2, 32, 32, 2], [68, 8, 8, 68, 68],[32, 2], [38, 38], [32, 19, 2],[53, 60, 44], [32, 17, 17, 2],[16, 16, 31, 31]);txt = getActiveGroup(gcbh);text(2, 100, txt,'verticalAlignment', 'top');
  w* trapezoidal4 : Subsystem  Tag=STV Subsys  LoadFcn=sigbuilder_block('load');  StartFcn=sigbuilder_block('start');  StopFcn=sigbuilder_block('stop');  ClipboardFcn=sigbuilder_block('clipboard');  mask(Sigbuilder block){tuvar=[0:10]}
      mask help: Simulink:masks:SigbuilderBlock_MD
      mask init:
      | if ~strcmp(get_param(bdroot(gcbh),'SimulationStatus'),'stopped') tuvar = sigbuilder_block('maskInit'); end
      settings: CopyFcn=sigbuilder_block('copy');  DeleteFcn=sigbuilder_block('delete');  ModelCloseFcn=sigbuilder_block('modelClose');  PreSaveFcn=sigbuilder_block('preSave');  PauseFcn=sigbuilder_block('pause');  ContinueFcn=sigbuilder_block('continue');  NameChangeFcn=sigbuilder_block('namechange');  OpenFcn=sigbuilder_block('open',[5.4 36 1141.2 516.6 ]);  CloseFcn=sigbuilder_block('close');
      mask Display: plot(0, 0, 100, 100,[2, 2, 32, 32, 2], [68, 8, 8, 68, 68],[32, 2], [38, 38], [32, 19, 2],[53, 60, 44], [32, 17, 17, 2],[16, 16, 31, 31]);txt = getActiveGroup(gcbh);text(2, 100, txt,'verticalAlignment', 'top');
  Out1 : Outport
  Out2 : Outport  Port=2
  Out3 : Outport  Port=3
  Out4 : Outport  Port=4
  wires:
  Sum5/1 -> Out3/1
  w* trapezoidal4/5(Signal 5) -> Sum6/5
  w* trapezoidal3/3(Signal 3) -> Sum5/3
  w* trapezoidal2/9(Signal 9) -> Sum4/9
  w* trapezoidal3/13(Signal 13) -> Sum5/13
  w* trapezoidal3/8(Signal 8) -> Sum5/8
  w* trapezoidal1/9(Signal 9) -> Sum3/9
  w* trapezoidal1/2(Signal 2) -> Sum3/2
  w* trapezoidal4/14(Signal 14) -> Sum6/14
  w* trapezoidal1/10(Signal 10) -> Sum3/10
  w* trapezoidal4/9(Signal 9) -> Sum6/9
  w* trapezoidal1/1(Signal 1) -> Sum3/1
  w* trapezoidal3/6(Signal 6) -> Sum5/6
  w* trapezoidal4/7(Signal 7) -> Sum6/7
  w* trapezoidal4/10(Signal 10) -> Sum6/10
  w* trapezoidal2/8(Signal 8) -> Sum4/8
  w* trapezoidal1/3(Signal 3) -> Sum3/3
  w* trapezoidal2/10(Signal 10) -> Sum4/10
  w* trapezoidal3/15(Signal 15) -> Sum5/15
  w* trapezoidal3/2(Signal 2) -> Sum5/2
  w* trapezoidal4/13(Signal 13) -> Sum6/13
  w* trapezoidal1/6(Signal 6) -> Sum3/6
  w* trapezoidal2/12(Signal 12) -> Sum4/12
  w* trapezoidal2/6(Signal 6) -> Sum4/6
  w* trapezoidal1/12(Signal 12) -> Sum3/12
  w* trapezoidal2/4(Signal 4) -> Sum4/4
  w* trapezoidal2/1(Signal 1) -> Sum4/1
  w* trapezoidal3/11(Signal 11) -> Sum5/11
  w* trapezoidal4/11(Signal 11) -> Sum6/11
  w* trapezoidal1/5(Signal 5) -> Sum3/5
  w* trapezoidal4/15(Signal 15) -> Sum6/15
  w* trapezoidal2/5(Signal 5) -> Sum4/5
  w* trapezoidal2/3(Signal 3) -> Sum4/3
  w* trapezoidal2/2(Signal 2) -> Sum4/2
  w* trapezoidal1/7(Signal 7) -> Sum3/7
  w* trapezoidal3/9(Signal 9) -> Sum5/9
  w* trapezoidal2/7(Signal 7) -> Sum4/7
  w* trapezoidal2/13(Signal 13) -> Sum4/13
  w* trapezoidal4/2(Signal 2) -> Sum6/2
  w* trapezoidal1/15(Signal 19) -> Sum3/15
  w* trapezoidal4/3(Signal 3) -> Sum6/3
  w* trapezoidal4/8(Signal 8) -> Sum6/8
  w* trapezoidal3/14(Signal 14) -> Sum5/14
  w* trapezoidal1/4(Signal 4) -> Sum3/4
  w* trapezoidal1/8(Signal 8) -> Sum3/8
  w* trapezoidal1/14(Signal 15) -> Sum3/14
  w* trapezoidal4/4(Signal 4) -> Sum6/4
  w* trapezoidal2/14(Signal 14) -> Sum4/15
  w* trapezoidal4/1(Signal 1) -> Sum6/1
  w* trapezoidal1/13(Signal 14) -> Sum3/13
  w* trapezoidal3/12(Signal 12) -> Sum5/12
  w* trapezoidal3/5(Signal 5) -> Sum5/5
  w* trapezoidal2/15(Signal 15) -> Sum4/14
  w* trapezoidal4/12(Signal 12) -> Sum6/12
  w* trapezoidal3/10(Signal 10) -> Sum5/10
  w* trapezoidal4/6(Signal 6) -> Sum6/6
  w* trapezoidal3/7(Signal 7) -> Sum5/7
  w* trapezoidal2/11(Signal 11) -> Sum4/11
  Sum3/1 -> Out1/1
  w* trapezoidal1/11(Signal 11) -> Sum3/11
  Sum6/1 -> Out4/1
  w* trapezoidal3/4(Signal 4) -> Sum5/4
  w* trapezoidal3/1(Signal 1) -> Sum5/1
  Sum4/1 -> Out2/1

== system diagrama_completo/Completo con w finito/w* trapezoidal ==
  Demux : Demux  Tag=STV Demux  Outputs=2
      settings: DisplayOption=none
  FromWs : FromWorkspace  Tag=STV FromWs  VariableName=tuvar
      SigBuilderData=|
      | common.afterFinalStr = 'Extrapolate'
      | common.sampleTime = 0
      | dataSet.timeRange = [0 25]
      | dataSet.name = 'Group 1'
      | sbobj.Groups.Name = 'Group 1'
      | sbobj.Groups.Signals(1).Name = 'Signal 1'
      | sbobj.Groups.Signals(1).XData = [0 5 5.2 9.8 10 25]
      | sbobj.Groups.Signals(1).YData = [0 0 1.25663706144 1.25663706144 0 0]
      | sbobj.Groups.Signals(2).Name = 'Signal 2'
      | sbobj.Groups.Signals(2).XData = [0 15 15.2 19.8 20 25]
      | sbobj.Groups.Signals(2).YData = [0 0 -1.25663706144 -1.25663706144 0 0]
      | sbobj.Groups.TimeRange = [0 25]
  Signal 1 : Outport  Tag=STV Outport
  Signal 2 : Outport  Tag=STV Outport  Port=2
  wires:
  FromWs/1 -> Demux/1
  Demux/1 -> Signal 1/1
  Demux/2 -> Signal 2/1

== system diagrama_completo/Completo con w infinito/Controlador de Movimiento ==
  w* : Inport
  w : Inport  Port=2
  Gain : Gain  Gain=ba
  Gain1 : Gain  Gain=ksa
  Gain2 : Gain  Gain=ksia
  Integrator : Integrator
  Integrator1 : Integrator
  Integrator2 : Integrator
  Sum : Sum  Inputs=|+++
  Sum1 : Sum  Inputs=|+-
  Theta* : Outport
  Tm*' : Outport  Port=2
  wires:
  w*/1 -> Integrator2/1, Sum1/1
  w/1 -> Sum1/2
  Sum1/1 -> Integrator/1, Gain/1  "ew"
  Sum/1 -> Tm*'/1
  Gain/1 -> Sum/3
  Gain1/1 -> Sum/2
  Integrator1/1 -> Gain2/1  "etheta/s"
  Integrator/1 -> Integrator1/1, Gain1/1  "etheta"
  Gain2/1 -> Sum/1
  Integrator2/1 -> Theta*/1  "etheta"

== system diagrama_completo/Completo con w infinito/Modulador de Torque ==
  T* : Inport
  Irqs : Inport  Port=2
  Irds : Inport  Port=3
  Ir0s : Inport  Port=4
  wm : Inport  Port=5
  Constant : Constant  Value=0
  Constant1 : Constant  Value=0
  Control de Corriente : Subsystem
  Gain3 : Gain  Gain=beq
  Gain9 : Gain  Gain=1/((3/2)*Pp*lambda_m)
  Sum : Sum  Inputs=|++
  vqs* : Outport
  vds* : Outport  Port=2
  v0s* : Outport  Port=3
  wires:
  Control de Corriente/2(vds*) -> vds*/1
  Irds/1 -> Control de Corriente/5(Irds)
  Gain9/1 -> Control de Corriente/1(Irqs*)
  Ir0s/1 -> Control de Corriente/6(Ir0s)
  Constant/1 -> Control de Corriente/3(Ir0s*)
  Control de Corriente/3(v0s*) -> v0s*/1
  Constant1/1 -> Control de Corriente/2(Irds*)
  Control de Corriente/1(vqs*) -> vqs*/1
  Irqs/1 -> Control de Corriente/4(Irqs)
  Sum/1 -> Gain9/1
  T*/1 -> Sum/1
  wm/1 -> Gain3/1, Control de Corriente/7(wm)
  Gain3/1 -> Sum/2

== system diagrama_completo/Completo con w infinito/Observador ==
  Tm : Inport
  thetam : Inport  Port=2
  Gain : Gain  Gain=kow
  Gain2 : Gain  Gain=kotheta
  Gain9 : Gain  Gain=1/Jeq
  Integrator : Integrator
  Integrator1 : Integrator
  Sum1 : Sum  Inputs=+|+
  Sum2 : Sum  Inputs=+|+
  Sum3 : Sum  Inputs=|+-
  wm_o : Outport
  theta_o : Outport  Port=2
  wires:
  Tm/1 -> Gain9/1
  Integrator1/1 -> theta_o/1, Sum3/2  "theta_o"
  Sum1/1 -> Integrator/1
  Sum2/1 -> wm_o/1, Integrator1/1
  thetam/1 -> Sum3/1
  Sum3/1 -> Gain2/1, Gain/1  "eo"
  Gain/1 -> Sum1/1
  Integrator/1 -> Sum2/2
  Gain2/1 -> Sum2/1
  Gain9/1 -> Sum1/2

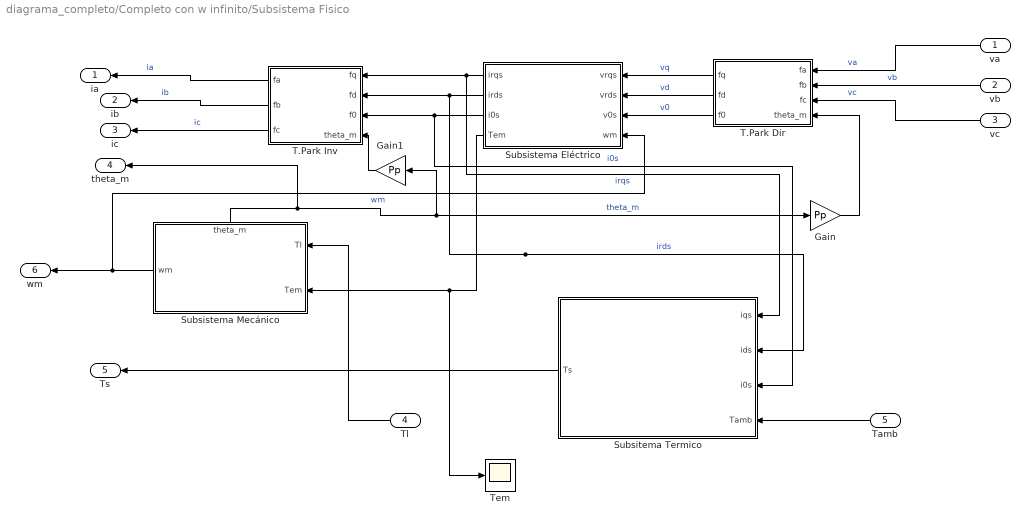
== system diagrama_completo/Completo con w infinito/Subsistema Fisico ==
  va : Inport
  vb : Inport  Port=2
  vc : Inport  Port=3
  Tl : Inport  Port=4
  Tamb : Inport  Port=5
  Gain : Gain  Gain=Pp
  Gain1 : Gain  Gain=Pp
  Subsistema Eléctrico : Subsystem
  Subsistema Mecánico : Subsystem
      settings: PortSchema="{\"entries\":[{\"content\":{\"sides\":[{\"content\":{\"connectorIds\":[\"In1\",\"In2\"]},\"type\":\"ConnectorPlacement.EquallySpacedRectSide\",\"uuid\":\"ee0e19e9-1195-452b-ab3d-8be3dd040414\"},{\"content\":{\"connectorIds\":[\"Out1\"],\"side\":\"RIGHT\"},\"type\":\"ConnectorPlacement.EquallySpacedRectSide\",\"uuid\":\"524e54e6-4967-4b42-ae12-58774e9397a0\"},{\"content\":{\"connectorIds\":[\"Out2\"],\"side\":\"TOP\"},\"type\":\"ConnectorPlacement.EquallySpacedRectSide\",\"uuid\":\"fab71378-68cb-4446-b02c-df48705d1789\"},{\"content\":{\"connectorIds\":[],\"side\":\"HIDDEN\"},\"type\":\"ConnectorPlacement.EquallySpacedRectSide\",\"uuid\":\"eea92cb8-3517-43ef-96fe-10b46f054d59\"}]},\"type\":\"ConnectorPlacement.EquallySpacedConnector\",\"uuid\":\"156d3ac5-e5c7-4248-8590-4f82c7370a76\"}],\"packageUris\":[\"http://schema.mathworks.com/mf0/Connector/R2020b\"],\"version\":\"1.0\"}"
  Subsitema Termico : Subsystem
  T.Park Dir : MATLAB Function  TreatAsAtomicUnit=on
  T.Park Inv : MATLAB Function  TreatAsAtomicUnit=on
  Tem : Scope
  ia : Outport
  ib : Outport  Port=2
  ic : Outport  Port=3
  theta_m : Outport  Port=4
  Ts : Outport  Port=5
  wm : Outport  Port=6
  wires:
  Subsitema Termico/1(Ts) -> Ts/1
  Tl/1 -> Subsistema Mecánico/1(Tl)
  T.Park Inv/3(fc) -> ic/1  "ic"
  vb/1 -> T.Park Dir/2(fb)  "vb"
  Tamb/1 -> Subsitema Termico/4(Tamb)
  T.Park Inv/1(fa) -> ia/1  "ia"
  Subsistema Mecánico/1(wm) -> Subsistema Eléctrico/4(wm), wm/1  "wm"
  T.Park Dir/1(fq) -> Subsistema Eléctrico/1(vrqs)  "vq"
  Subsistema Eléctrico/3(i0s) -> Subsitema Termico/3(i0s), T.Park Inv/3(f0)  "i0s"
  Subsistema Eléctrico/1(irqs) -> Subsitema Termico/1(iqs), T.Park Inv/1(fq)  "irqs"
  Subsistema Eléctrico/2(irds) -> Subsitema Termico/2(ids), T.Park Inv/2(fd)  "irds"
  T.Park Dir/3(f0) -> Subsistema Eléctrico/3(v0s)  "v0"
  T.Park Dir/2(fd) -> Subsistema Eléctrico/2(vrds)  "vd"
  vc/1 -> T.Park Dir/3(fc)  "vc"
  T.Park Inv/2(fb) -> ib/1  "ib"
  Subsistema Mecánico/2(theta_m) -> theta_m/1, Gain1/1, Gain/1  "theta_m"
  va/1 -> T.Park Dir/1(fa)  "va"
  Subsistema Eléctrico/4(Tem) -> Tem/1, Subsistema Mecánico/2(Tem)
  Gain/1 -> T.Park Dir/4(theta_m)
  Gain1/1 -> T.Park Inv/4(theta_m)

== system diagrama_completo/Completo con w infinito/Tl* ==
  Demux : Demux  Tag=STV Demux  Outputs=1
      settings: DisplayOption=none
  FromWs : FromWorkspace  Tag=STV FromWs  VariableName=tuvar
      SigBuilderData=|
      | common.afterFinalStr = 'Extrapolate'
      | common.sampleTime = 0
      | dataSet.timeRange = [0 25]
      | dataSet.name = 'Group 1'
      | sbobj.Groups.Name = 'Group 1'
      | sbobj.Groups.Signals.Name = 'Signal 1'
      | sbobj.Groups.Signals.XData = [0 1 1 25]
      | sbobj.Groups.Signals.YData = [0 0 6.28 6.28]
      | sbobj.Groups.TimeRange = [0 25]
  Signal 1 : Outport  Tag=STV Outport
  wires:
  Demux/1 -> Signal 1/1
  FromWs/1 -> Demux/1

== system diagrama_completo/Completo con w infinito/w* cuadrada ==
  Demux : Demux  Tag=STV Demux  Outputs=2
      settings: DisplayOption=none
  FromWs : FromWorkspace  Tag=STV FromWs  VariableName=tuvar
      SigBuilderData=|
      | common.afterFinalStr = 'Extrapolate'
      | common.sampleTime = 0
      | dataSet.timeRange = [0 25]
      | dataSet.name = 'Group 1'
      | sbobj.Groups.Name = 'Group 1'
      | sbobj.Groups.Signals(1).Name = 'Signal 1'
      | sbobj.Groups.Signals(1).XData = [0 5 5 10 10 25]
      | sbobj.Groups.Signals(1).YData = [0 0 1.25663706144 1.25663706144 0 0]
      | sbobj.Groups.Signals(2).Name = 'Signal 2'
      | sbobj.Groups.Signals(2).XData = [0 15 15 20 20 25]
      | sbobj.Groups.Signals(2).YData = [0 0 -1.25663706144 -1.25663706144 0 0]
      | sbobj.Groups.TimeRange = [0 25]
  Signal 1 : Outport  Tag=STV Outport
  Signal 2 : Outport  Tag=STV Outport  Port=2
  wires:
  FromWs/1 -> Demux/1
  Demux/1 -> Signal 1/1
  Demux/2 -> Signal 2/1

== system diagrama_completo/Completo con w infinito/w* p//600 s ==
  Sum{3..6} (4 alike) : Sum  Inputs=|+++++++++++++++
  w* trapezoidal1 : Subsystem  Tag=STV Subsys  LoadFcn=sigbuilder_block('load');  StartFcn=sigbuilder_block('start');  StopFcn=sigbuilder_block('stop');  ClipboardFcn=sigbuilder_block('clipboard');  mask(Sigbuilder block){tuvar=[0:10]}
      mask help: Simulink:masks:SigbuilderBlock_MD
      mask init:
      | if ~strcmp(get_param(bdroot(gcbh),'SimulationStatus'),'stopped') tuvar = sigbuilder_block('maskInit'); end
      settings: CopyFcn=sigbuilder_block('copy');  DeleteFcn=sigbuilder_block('delete');  ModelCloseFcn=sigbuilder_block('modelClose');  PreSaveFcn=sigbuilder_block('preSave');  PauseFcn=sigbuilder_block('pause');  ContinueFcn=sigbuilder_block('continue');  NameChangeFcn=sigbuilder_block('namechange');  OpenFcn=sigbuilder_block('open',[5.4 36 1141.2 516.6 ]);  CloseFcn=sigbuilder_block('close');
      mask Display: plot(0, 0, 100, 100,[2, 2, 32, 32, 2], [68, 8, 8, 68, 68],[32, 2], [38, 38], [32, 19, 2],[53, 60, 44], [32, 17, 17, 2],[16, 16, 31, 31]);txt = getActiveGroup(gcbh);text(2, 100, txt,'verticalAlignment', 'top');
  w* trapezoidal2 : Subsystem  Tag=STV Subsys  LoadFcn=sigbuilder_block('load');  StartFcn=sigbuilder_block('start');  StopFcn=sigbuilder_block('stop');  ClipboardFcn=sigbuilder_block('clipboard');  mask(Sigbuilder block){tuvar=[0:10]}
      mask help: Simulink:masks:SigbuilderBlock_MD
      mask init:
      | if ~strcmp(get_param(bdroot(gcbh),'SimulationStatus'),'stopped') tuvar = sigbuilder_block('maskInit'); end
      settings: CopyFcn=sigbuilder_block('copy');  DeleteFcn=sigbuilder_block('delete');  ModelCloseFcn=sigbuilder_block('modelClose');  PreSaveFcn=sigbuilder_block('preSave');  PauseFcn=sigbuilder_block('pause');  ContinueFcn=sigbuilder_block('continue');  NameChangeFcn=sigbuilder_block('namechange');  OpenFcn=sigbuilder_block('open',[5.4 36 1141.2 516.6 ]);  CloseFcn=sigbuilder_block('close');
      mask Display: plot(0, 0, 100, 100,[2, 2, 32, 32, 2], [68, 8, 8, 68, 68],[32, 2], [38, 38], [32, 19, 2],[53, 60, 44], [32, 17, 17, 2],[16, 16, 31, 31]);txt = getActiveGroup(gcbh);text(2, 100, txt,'verticalAlignment', 'top');
  w* trapezoidal3 : Subsystem  Tag=STV Subsys  LoadFcn=sigbuilder_block('load');  StartFcn=sigbuilder_block('start');  StopFcn=sigbuilder_block('stop');  ClipboardFcn=sigbuilder_block('clipboard');  mask(Sigbuilder block){tuvar=[0:10]}
      mask help: Simulink:masks:SigbuilderBlock_MD
      mask init:
      | if ~strcmp(get_param(bdroot(gcbh),'SimulationStatus'),'stopped') tuvar = sigbuilder_block('maskInit'); end
      settings: CopyFcn=sigbuilder_block('copy');  DeleteFcn=sigbuilder_block('delete');  ModelCloseFcn=sigbuilder_block('modelClose');  PreSaveFcn=sigbuilder_block('preSave');  PauseFcn=sigbuilder_block('pause');  ContinueFcn=sigbuilder_block('continue');  NameChangeFcn=sigbuilder_block('namechange');  OpenFcn=sigbuilder_block('open',[5.4 36 1141.2 516.6 ]);  CloseFcn=sigbuilder_block('close');
      mask Display: plot(0, 0, 100, 100,[2, 2, 32, 32, 2], [68, 8, 8, 68, 68],[32, 2], [38, 38], [32, 19, 2],[53, 60, 44], [32, 17, 17, 2],[16, 16, 31, 31]);txt = getActiveGroup(gcbh);text(2, 100, txt,'verticalAlignment', 'top');
  w* trapezoidal4 : Subsystem  Tag=STV Subsys  LoadFcn=sigbuilder_block('load');  StartFcn=sigbuilder_block('start');  StopFcn=sigbuilder_block('stop');  ClipboardFcn=sigbuilder_block('clipboard');  mask(Sigbuilder block){tuvar=[0:10]}
      mask help: Simulink:masks:SigbuilderBlock_MD
      mask init:
      | if ~strcmp(get_param(bdroot(gcbh),'SimulationStatus'),'stopped') tuvar = sigbuilder_block('maskInit'); end
      settings: CopyFcn=sigbuilder_block('copy');  DeleteFcn=sigbuilder_block('delete');  ModelCloseFcn=sigbuilder_block('modelClose');  PreSaveFcn=sigbuilder_block('preSave');  PauseFcn=sigbuilder_block('pause');  ContinueFcn=sigbuilder_block('continue');  NameChangeFcn=sigbuilder_block('namechange');  OpenFcn=sigbuilder_block('open',[5.4 36 1141.2 516.6 ]);  CloseFcn=sigbuilder_block('close');
      mask Display: plot(0, 0, 100, 100,[2, 2, 32, 32, 2], [68, 8, 8, 68, 68],[32, 2], [38, 38], [32, 19, 2],[53, 60, 44], [32, 17, 17, 2],[16, 16, 31, 31]);txt = getActiveGroup(gcbh);text(2, 100, txt,'verticalAlignment', 'top');
  Out1 : Outport
  Out2 : Outport  Port=2
  Out3 : Outport  Port=3
  Out4 : Outport  Port=4
  wires:
  Sum5/1 -> Out3/1
  w* trapezoidal4/5(Signal 5) -> Sum6/5
  w* trapezoidal3/3(Signal 3) -> Sum5/3
  w* trapezoidal2/9(Signal 9) -> Sum4/9
  w* trapezoidal3/13(Signal 13) -> Sum5/13
  w* trapezoidal3/8(Signal 8) -> Sum5/8
  w* trapezoidal1/9(Signal 9) -> Sum3/9
  w* trapezoidal1/2(Signal 2) -> Sum3/2
  w* trapezoidal4/14(Signal 14) -> Sum6/14
  w* trapezoidal1/10(Signal 10) -> Sum3/10
  w* trapezoidal4/9(Signal 9) -> Sum6/9
  w* trapezoidal1/1(Signal 1) -> Sum3/1
  w* trapezoidal3/6(Signal 6) -> Sum5/6
  w* trapezoidal4/7(Signal 7) -> Sum6/7
  w* trapezoidal4/10(Signal 10) -> Sum6/10
  w* trapezoidal2/8(Signal 8) -> Sum4/8
  w* trapezoidal1/3(Signal 3) -> Sum3/3
  w* trapezoidal2/10(Signal 10) -> Sum4/10
  w* trapezoidal3/15(Signal 15) -> Sum5/15
  w* trapezoidal3/2(Signal 2) -> Sum5/2
  w* trapezoidal4/13(Signal 13) -> Sum6/13
  w* trapezoidal1/6(Signal 6) -> Sum3/6
  w* trapezoidal2/12(Signal 12) -> Sum4/12
  w* trapezoidal2/6(Signal 6) -> Sum4/6
  w* trapezoidal1/12(Signal 12) -> Sum3/12
  w* trapezoidal2/4(Signal 4) -> Sum4/4
  w* trapezoidal2/1(Signal 1) -> Sum4/1
  w* trapezoidal3/11(Signal 11) -> Sum5/11
  w* trapezoidal4/11(Signal 11) -> Sum6/11
  w* trapezoidal1/5(Signal 5) -> Sum3/5
  w* trapezoidal4/15(Signal 15) -> Sum6/15
  w* trapezoidal2/5(Signal 5) -> Sum4/5
  w* trapezoidal2/3(Signal 3) -> Sum4/3
  w* trapezoidal2/2(Signal 2) -> Sum4/2
  w* trapezoidal1/7(Signal 7) -> Sum3/7
  w* trapezoidal3/9(Signal 9) -> Sum5/9
  w* trapezoidal2/7(Signal 7) -> Sum4/7
  w* trapezoidal2/13(Signal 13) -> Sum4/13
  w* trapezoidal4/2(Signal 2) -> Sum6/2
  w* trapezoidal1/15(Signal 19) -> Sum3/15
  w* trapezoidal4/3(Signal 3) -> Sum6/3
  w* trapezoidal4/8(Signal 8) -> Sum6/8
  w* trapezoidal3/14(Signal 14) -> Sum5/14
  w* trapezoidal1/4(Signal 4) -> Sum3/4
  w* trapezoidal1/8(Signal 8) -> Sum3/8
  w* trapezoidal1/14(Signal 15) -> Sum3/14
  w* trapezoidal4/4(Signal 4) -> Sum6/4
  w* trapezoidal2/14(Signal 14) -> Sum4/15
  w* trapezoidal4/1(Signal 1) -> Sum6/1
  w* trapezoidal1/13(Signal 14) -> Sum3/13
  w* trapezoidal3/12(Signal 12) -> Sum5/12
  w* trapezoidal3/5(Signal 5) -> Sum5/5
  w* trapezoidal2/15(Signal 15) -> Sum4/14
  w* trapezoidal4/12(Signal 12) -> Sum6/12
  w* trapezoidal3/10(Signal 10) -> Sum5/10
  w* trapezoidal4/6(Signal 6) -> Sum6/6
  w* trapezoidal3/7(Signal 7) -> Sum5/7
  w* trapezoidal2/11(Signal 11) -> Sum4/11
  Sum3/1 -> Out1/1
  w* trapezoidal1/11(Signal 11) -> Sum3/11
  Sum6/1 -> Out4/1
  w* trapezoidal3/4(Signal 4) -> Sum5/4
  w* trapezoidal3/1(Signal 1) -> Sum5/1
  Sum4/1 -> Out2/1

== system diagrama_completo/Completo con w infinito/w* trapezoidal ==
  Demux : Demux  Tag=STV Demux  Outputs=2
      settings: DisplayOption=none
  FromWs : FromWorkspace  Tag=STV FromWs  VariableName=tuvar
      SigBuilderData=|
      | common.afterFinalStr = 'Extrapolate'
      | common.sampleTime = 0
      | dataSet.timeRange = [0 25]
      | dataSet.name = 'Group 1'
      | sbobj.Groups.Name = 'Group 1'
      | sbobj.Groups.Signals(1).Name = 'Signal 1'
      | sbobj.Groups.Signals(1).XData = [0 5 5.2 9.8 10 25]
      | sbobj.Groups.Signals(1).YData = [0 0 1.25663706144 1.25663706144 0 0]
      | sbobj.Groups.Signals(2).Name = 'Signal 2'
      | sbobj.Groups.Signals(2).XData = [0 15 15.2 19.8 20 25]
      | sbobj.Groups.Signals(2).YData = [0 0 -1.25663706144 -1.25663706144 0 0]
      | sbobj.Groups.TimeRange = [0 25]
  Signal 1 : Outport  Tag=STV Outport
  Signal 2 : Outport  Tag=STV Outport  Port=2
  wires:
  FromWs/1 -> Demux/1
  Demux/1 -> Signal 1/1
  Demux/2 -> Signal 2/1

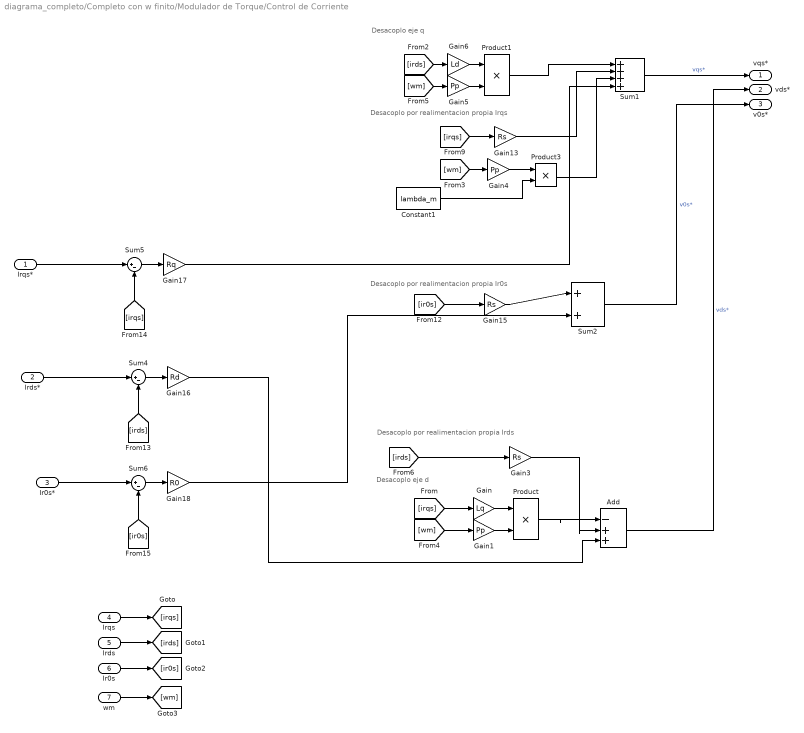
== system diagrama_completo/Completo con w finito/Modulador de Torque/Control de Corriente ==
  note: Desacoplo por realimentacion propia Ir0s
  note: Desacoplo por realimentacion propia Irqs
  note: Desacoplo por realimentacion propia Irds
  note: Desacoplo eje d
  note: Desacoplo eje q
  Irqs* : Inport
  Irds* : Inport  Port=2
  Ir0s* : Inport  Port=3
  Irqs : Inport  Port=4
  Irds : Inport  Port=5
  Ir0s : Inport  Port=6
  wm : Inport  Port=7
  Add : Sum  Inputs=|-++
  Constant1 : Constant  Value=lambda_m
  Gain : Gain  Gain=Lq
  Gain1 : Gain  Gain=Pp
  Gain13 : Gain  Gain=Rs
  Gain15 : Gain  Gain=Rs
  Gain16 : Gain  Gain=Rd
  Gain17 : Gain  Gain=Rq
  Gain18 : Gain  Gain=R0
  Gain3 : Gain  Gain=Rs
  Gain4 : Gain  Gain=Pp
  Gain5 : Gain  Gain=Pp
  Gain6 : Gain  Gain=Ld
  Product : Product
  Product1 : Product
  Product3 : Product
  Sum1 : Sum  Inputs=|++++
  Sum2 : Sum  Inputs=|++
  Sum4 : Sum  Inputs=|+-
  Sum5 : Sum  Inputs=|+-
  Sum6 : Sum  Inputs=|+-
  vqs* : Outport
  vds* : Outport  Port=2
  v0s* : Outport  Port=3
  wires:
  [ir0s] -> Sum6/2
  Sum2/1 -> v0s*/1  "v0s*"
  Irqs*/1 -> Sum5/1
  Ir0s*/1 -> Sum6/1
  Gain3/1 -> Add/2
  [irqs] -> Gain13/1
  [irds] -> Sum4/2
  [ir0s] -> Gain15/1
  Sum5/1 -> Gain17/1
  [irqs] -> Sum5/2
  [irds] -> Gain3/1
  Gain13/1 -> Sum1/2
  Sum6/1 -> Gain18/1
  Irds*/1 -> Sum4/1
  Gain15/1 -> Sum2/1
  Gain18/1 -> Sum2/2
  Gain17/1 -> Sum1/4
  Product1/1 -> Sum1/1
  Product/1 -> Add/1
  Gain5/1 -> Product1/2
  Gain/1 -> Product/1
  Gain4/1 -> Product3/1
  Sum4/1 -> Gain16/1
  Constant1/1 -> Product3/2
  Product3/1 -> Sum1/3
  Add/1 -> vds*/1  "vds*"
  Sum1/1 -> vqs*/1  "vqs*"
  Irqs/1 -> [irqs]
  Irds/1 -> [irds]
  Ir0s/1 -> [ir0s]
  [irqs] -> Gain/1
  Gain1/1 -> Product/2
  [wm] -> Gain1/1
  wm/1 -> [wm]
  [wm] -> Gain4/1
  [wm] -> Gain5/1
  [irds] -> Gain6/1
  Gain6/1 -> Product1/1
  Gain16/1 -> Add/3
